simulink model "SingleTrack5states"  (R2018a)
settings: Solver=ode4  StartTime=0.0  StopTime=200  FixedStep=.001  MaxStep=0.001  MinStep=0.0001  RelTol=1e-1
values from neighbouring files (symbols this model uses):
  df_max = 0.35    [init_model.m]
  dr_max = 0    [init_model.m]
  initBeta = 0    [init_model.m]
  initR = 0    [init_model.m]
  initV = 10    [init_model.m]
  omegaR_max = 200    [init_model.m]
undefined symbols (not defined in the file or in its folder): car
settings Model: Creator=efrem  LastModifiedBy=efrem
settings SolverCC: ZeroCrossAlgorithm=Adaptive  AlgebraicLoopSolver=LineSearch
settings DebuggingCC: MaxConsecutiveZCsMsg=none
settings CodeAppCC: StateflowObjectComments=on

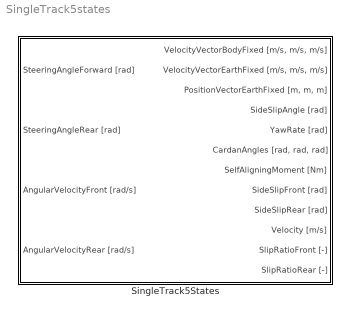
== system SingleTrack5states ==
  SingleTrack5States : Subsystem

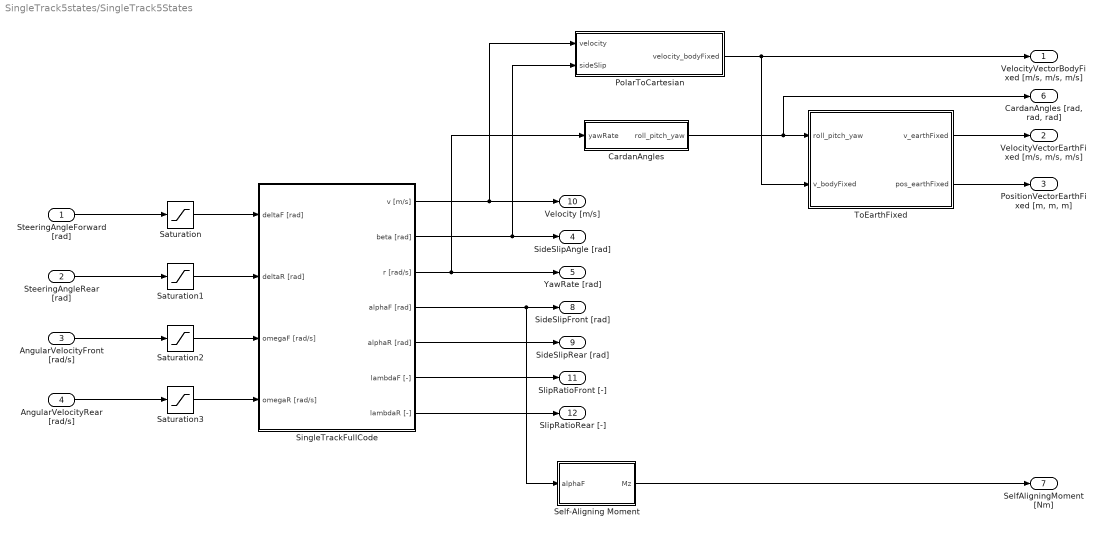
== system SingleTrack5states/SingleTrack5States ==
  SteeringAngleForward [rad] : Inport
  SteeringAngleRear [rad] : Inport  Port=2
  AngularVelocityFront [rad/s] : Inport  Port=3
  AngularVelocityRear [rad/s] : Inport  Port=4
  CardanAngles : Subsystem
  PolarToCartesian : Subsystem
  Saturation : Saturate  UpperLimit=df_max  LowerLimit=-df_max  ZeroCross=off
  Saturation1 : Saturate  UpperLimit=dr_max  LowerLimit=-dr_max  ZeroCross=off
  Saturation2 : Saturate  UpperLimit=omegaR_max  LowerLimit=0  ZeroCross=off
  Saturation3 : Saturate  UpperLimit=omegaR_max  LowerLimit=0  ZeroCross=off
  Self-Aligning Moment : Subsystem
  SingleTrackFullCode : Subsystem
  ToEarthFixed : Subsystem
  "VelocityVectorBodyFixed [m/s, m/s, m/s]" : Outport
  "VelocityVectorEarthFixed [m/s, m/s, m/s]" : Outport  Port=2
  "PositionVectorEarthFixed [m, m, m]" : Outport  Port=3
  SideSlipAngle [rad] : Outport  Port=4
  YawRate [rad] : Outport  Port=5
  "CardanAngles [rad, rad, rad]" : Outport  Port=6
  SelfAligningMoment [Nm] : Outport  Port=7
  SideSlipFront [rad] : Outport  Port=8
  SideSlipRear [rad] : Outport  Port=9
  Velocity [m/s] : Outport  Port=10
  SlipRatioFront [-] : Outport  Port=11
  SlipRatioRear [-] : Outport  Port=12
  wires:
  SingleTrackFullCode/3(r [rad/s]) -> CardanAngles/1(yawRate), YawRate [rad]/1
  ToEarthFixed/2(pos_earthFixed) -> "PositionVectorEarthFixed [m, m, m]"/1
  Self-Aligning Moment/1(Mz) -> SelfAligningMoment [Nm]/1
  PolarToCartesian/1(velocity_bodyFixed) -> ToEarthFixed/2(v_bodyFixed), "VelocityVectorBodyFixed [m/s, m/s, m/s]"/1
  SingleTrackFullCode/2(beta [rad]) -> PolarToCartesian/2(sideSlip), SideSlipAngle [rad]/1
  ToEarthFixed/1(v_earthFixed) -> "VelocityVectorEarthFixed [m/s, m/s, m/s]"/1
  CardanAngles/1(roll_pitch_yaw) -> ToEarthFixed/1(roll_pitch_yaw), "CardanAngles [rad, rad, rad]"/1
  SteeringAngleForward [rad]/1 -> Saturation/1
  AngularVelocityFront [rad/s]/1 -> Saturation2/1
  AngularVelocityRear [rad/s]/1 -> Saturation3/1
  Saturation1/1 -> SingleTrackFullCode/2(deltaR [rad])
  Saturation2/1 -> SingleTrackFullCode/3(omegaF [rad/s])
  Saturation3/1 -> SingleTrackFullCode/4(omegaR [rad/s])
  SteeringAngleRear [rad]/1 -> Saturation1/1
  SingleTrackFullCode/1(v [m/s]) -> PolarToCartesian/1(velocity), Velocity [m/s]/1
  Saturation/1 -> SingleTrackFullCode/1(deltaF [rad])
  SingleTrackFullCode/4(alphaF [rad]) -> Self-Aligning Moment/1(alphaF), SideSlipFront [rad]/1
  SingleTrackFullCode/5(alphaR [rad]) -> SideSlipRear [rad]/1
  SingleTrackFullCode/6(lambdaF [-]) -> SlipRatioFront [-]/1
  SingleTrackFullCode/7(lambdaR [-]) -> SlipRatioRear [-]/1

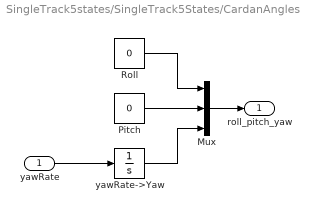
== system SingleTrack5states/SingleTrack5States/CardanAngles ==
  yawRate : Inport
  Mux : Mux  Inputs=3
  Pitch : Constant  Value=0
  Roll : Constant  Value=0
  yawRate->Yaw : Integrator
  roll_pitch_yaw : Outport
  wires:
  Pitch/1 -> Mux/2
  Roll/1 -> Mux/1
  Mux/1 -> roll_pitch_yaw/1
  yawRate->Yaw/1 -> Mux/3
  yawRate/1 -> yawRate->Yaw/1

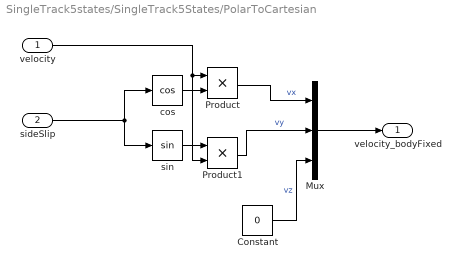
== system SingleTrack5states/SingleTrack5States/PolarToCartesian ==
  velocity : Inport
  sideSlip : Inport  Port=2
  Constant : Constant  Value=0
  Mux : Mux  Inputs=3
  Product : Product
  Product1 : Product
  cos : Trigonometry  Operator=cos
  sin : Trigonometry
  velocity_bodyFixed : Outport
  wires:
  Product/1 -> Mux/1  "vx"
  velocity/1 -> Product/1, Product1/2
  sin/1 -> Product1/1
  sideSlip/1 -> cos/1, sin/1
  Product1/1 -> Mux/2  "vy"
  cos/1 -> Product/2
  Constant/1 -> Mux/3  "vz"
  Mux/1 -> velocity_bodyFixed/1

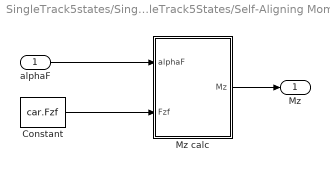
== system SingleTrack5states/SingleTrack5States/Self-Aligning Moment ==
  alphaF : Inport
  Constant : Constant  Value=car.Fzf
  Mz calc : MATLAB Function  TreatAsAtomicUnit=on
  Mz : Outport
  wires:
  Mz calc/1(Mz) -> Mz/1
  Constant/1 -> Mz calc/2(Fzf)
  alphaF/1 -> Mz calc/1(alphaF)

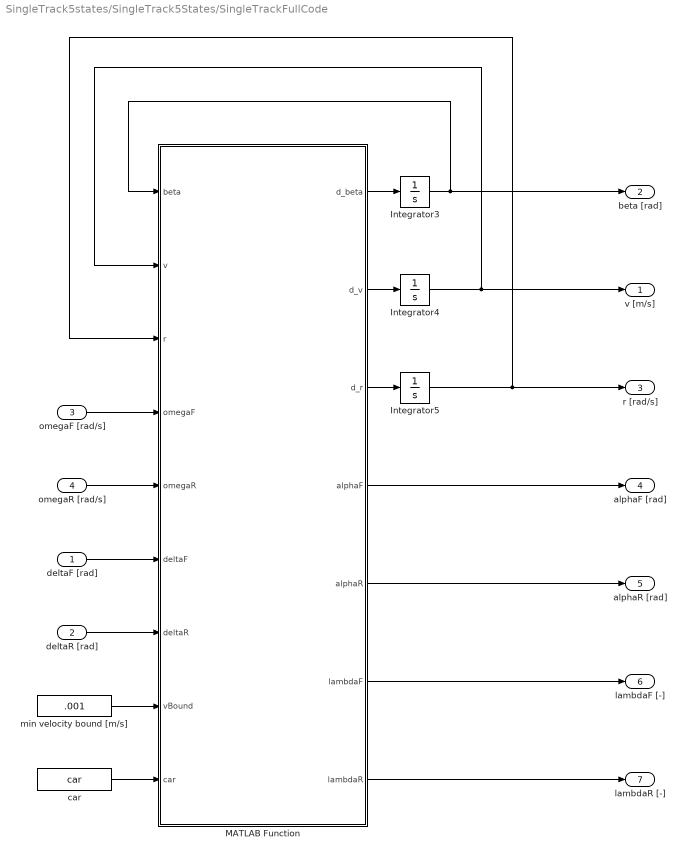
== system SingleTrack5states/SingleTrack5States/SingleTrackFullCode ==
  deltaF [rad] : Inport
  deltaR [rad] : Inport  Port=2
  omegaF [rad/s] : Inport  Port=3
  omegaR [rad/s] : Inport  Port=4
  Integrator3 : Integrator  InitialCondition=initBeta  UpperSaturationLimit=pi/2  LowerSaturationLimit=-pi/2  ZeroCross=off
  Integrator4 : Integrator  InitialCondition=initV  UpperSaturationLimit=pi/2  LowerSaturationLimit=-pi/2  ZeroCross=off
  Integrator5 : Integrator  InitialCondition=initR  UpperSaturationLimit=pi/2  LowerSaturationLimit=-pi/2  ZeroCross=off
  MATLAB Function : MATLAB Function  TreatAsAtomicUnit=on
  car : Constant  Value=car  OutDataTypeStr=Bus: car_bus
  min velocity bound [m/s] : Constant  Value=.001
  v [m/s] : Outport
  beta [rad] : Outport  Port=2
  r [rad/s] : Outport  Port=3
  alphaF [rad] : Outport  Port=4
  alphaR [rad] : Outport  Port=5
  lambdaF [-] : Outport  Port=6
  lambdaR [-] : Outport  Port=7
  wires:
  car/1 -> MATLAB Function/9(car)
  min velocity bound [m/s]/1 -> MATLAB Function/8(vBound)
  MATLAB Function/1(d_beta) -> Integrator3/1
  Integrator3/1 -> MATLAB Function/1(beta), beta [rad]/1
  MATLAB Function/2(d_v) -> Integrator4/1
  Integrator4/1 -> MATLAB Function/2(v), v [m/s]/1
  MATLAB Function/3(d_r) -> Integrator5/1
  Integrator5/1 -> MATLAB Function/3(r), r [rad/s]/1
  MATLAB Function/4(alphaF) -> alphaF [rad]/1
  MATLAB Function/5(alphaR) -> alphaR [rad]/1
  MATLAB Function/6(lambdaF) -> lambdaF [-]/1
  MATLAB Function/7(lambdaR) -> lambdaR [-]/1
  deltaF [rad]/1 -> MATLAB Function/6(deltaF)
  deltaR [rad]/1 -> MATLAB Function/7(deltaR)
  omegaF [rad/s]/1 -> MATLAB Function/4(omegaF)
  omegaR [rad/s]/1 -> MATLAB Function/5(omegaR)

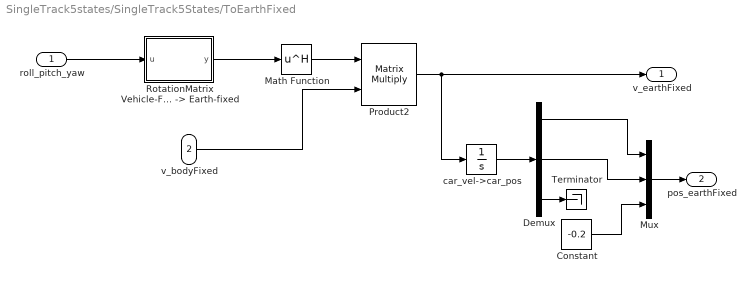
== system SingleTrack5states/SingleTrack5States/ToEarthFixed ==
  roll_pitch_yaw : Inport
  v_bodyFixed : Inport  Port=2
  Constant : Constant  Value=-0.2
  Demux : Demux  Outputs=3
  Math Function : Math  Operator=hermitian  SaturateOnIntegerOverflow=on
  Mux : Mux  Inputs=3
  Product2 : Product  Multiplication=Matrix(*)
  "RotationMatrix Vehicle-Fixed -> Earth-fixed" : MATLAB Function  TreatAsAtomicUnit=on
  Terminator : Terminator
  car_vel->car_pos : Integrator
  v_earthFixed : Outport
  pos_earthFixed : Outport  Port=2
  wires:
  v_bodyFixed/1 -> Product2/2
  Product2/1 -> v_earthFixed/1, car_vel->car_pos/1
  Constant/1 -> Mux/3
  Mux/1 -> pos_earthFixed/1
  car_vel->car_pos/1 -> Demux/1
  Demux/2 -> Mux/2
  Demux/1 -> Mux/1
  Math Function/1 -> Product2/1
  roll_pitch_yaw/1 -> "RotationMatrix Vehicle-Fixed -> Earth-fixed"/1(u)
  "RotationMatrix Vehicle-Fixed -> Earth-fixed"/1(y) -> Math Function/1
  Demux/3 -> Terminator/1

== matlab function SingleTrack5states/SingleTrack5States/ToEarthFixed/RotationMatrix Vehicle-Fixed -> Earth-fixed ==
  data: u input; y output
function y = fcn(u)

phi   = u(1); %roll
theta = u(2); %pitch
psi   = u(3); %yaw

% transformation matrix from the Earth-fixed to the vehicle-fixed
% coordinate frames
ETV = [cos(theta)*cos(psi),   sin(phi)*sin(theta)*cos(psi) - cos(phi)*sin(psi),   cos(phi)*sin(theta)*cos(psi) + sin(phi)*sin(psi);
       cos(theta)*sin(psi),   sin(phi)*sin(theta)*sin(psi) + cos(phi)*cos(psi),   cos(phi)*sin(theta)*sin(psi) - sin(phi)*cos(psi);
               -sin(theta),                                sin(phi)*cos(theta),                                cos(phi)*cos(theta)];
         
y = ETV';

== matlab function SingleTrack5states/SingleTrack5States/Self-Aligning Moment/Mz calc ==
  data: alphaF input; Mz output; Fzf input
function Mz = fcn(alphaF, Fzf)
    alphaF = rad2deg(alphaF);
    
    Bz = .15;
    Cz = 2.3;
    Dz = -.05 * Fzf;
    Ez = -10;
    
    Mz = Dz*sin((Cz*atan(Bz*alphaF - Ez*(Bz*alphaF - atan(Bz*alphaF)))));
end

== matlab function SingleTrack5states/SingleTrack5States/SingleTrackFullCode/MATLAB Function ==
  data: beta input; v input; r input; d_beta output; d_v output; d_r output; omegaF input; omegaR input; deltaF input; deltaR input; vBound input; car input; alphaF output; alphaR output; lambdaF output; lambdaR output
function [d_beta, d_v, d_r, alphaF, alphaR, lambdaF, lambdaR]= SingleTrackModel(beta, v, r, omegaF, omegaR, deltaF, deltaR, vBound, car)

    %% Parse Parameters 
    lf  = car.lf;
    lr  = car.lr;
    m   = car.m;
    Fzf = car.Fzf;
    Fzr = car.Fzr;
    p   = car.p;
    I   = car.I;
    
    Cdy = car.Tire.Cdy;
    Cby = car.Tire.Cby;
    Ccy = car.Tire.Ccy;
    Cey = car.Tire.Cey;
    Cdx = car.Tire.Cdx;
    Cbx = car.Tire.Cbx;
    Ccx = car.Tire.Ccx;
    Cex = car.Tire.Cex;
    
    %% Apply Deadzone for the Velocity (due to division by zero)
    if(v < vBound && v >= 0) 
		v = v+vBound;
	elseif (v > -vBound && v <0)
        v = v-vBound;
    end
    
    %% Wheel Kinematics
    vf = [cos(deltaF) sin(deltaF); -sin(deltaF) cos(deltaF)]*...
         [v*cos(beta); v*sin(beta) + lf*r];
    vr = [cos(deltaR) sin(deltaR); -sin(deltaR) cos(deltaR)]*...
         [v*cos(beta); v*sin(beta) - lr*r];
    vxf = vf(1);
    vyf = vf(2);
    vxr = vr(1);
    vyr = vr(2); 
    
    % slip angles of tires
    alphaF = -atan2(vyf, abs(vxf));
    alphaR = -atan2(vyr, abs(vxr));
     
    %% Slip Ratios
    lambdaF = (omegaF*p - vxf)/max(abs(omegaF*p), abs(vxf));
    lambdaR = (omegaR*p - vxr)/max(abs(omegaR*p), abs(vxr));
    
    lambdaF(lambdaF > 1)  = 1;
    lambdaF(lambdaF < -1) = -1;
    lambdaR(lambdaR > 1)  = 1;
    lambdaR(lambdaR < -1) = -1;
    
    %% Tire Models
    Fyf0 = Cdy * Fzf * sin(Ccy * atan(Cby*alphaF - Cey*(Cby*alphaF - atan(Cby*alphaF))));
    Fyr0 = Cdy * Fzr * sin(Ccy * atan(Cby*alphaR - Cey*(Cby*alphaR - atan(Cby*alphaR))));

    Fxf0 = Cdx * Fzf * sin(Ccx * atan(Cbx*lambdaF - Cex*(Cbx*lambdaF - atan(Cbx*lambdaF))));
    Fxr0 = Cdx * Fzr * sin(Ccx * atan(Cbx*lambdaR - Cex*(Cbx*lambdaR - atan(Cbx*lambdaR))));
    
    %% Traction Ellipse Front
    betaStar = acos(abs(lambdaF)/sqrt(lambdaF^2 + sin(alphaF)^2));

    mu_x_act = Fxf0/Fzf;
    mu_y_act = Fyf0/Fzf;

    mu_x_max = Cdx;
    mu_y_max = Cdy;

    mu_x = 1/sqrt((1/mu_x_act)^2 + (tan(betaStar)/mu_y_max)^2);
    mu_y = tan(betaStar)/sqrt((1/mu_x_max)^2 + (tan(betaStar)/mu_y_act)^2);

    Fxf = abs(mu_x/mu_x_act)*Fxf0;
    Fyf = abs(mu_y/mu_y_act)*Fyf0;

    if isnan(Fxf)
        Fxf = 0;
    end

    if isnan(Fyf)
        Fyf = 0;
    end

    if Fzf == 0
        Fxf = Fxf0;
        Fyf = Fyf0;
    end
    
    %% Traction Ellipse Rear
    betaStar = acos(abs(lambdaR)/sqrt(lambdaR^2 + sin(alphaR)^2));

    mu_x_act = Fxr0/Fzr;
    mu_y_act = Fyr0/Fzr;

    mu_x_max = Cdx;
    mu_y_max = Cdy;

    mu_x = 1/sqrt((1/mu_x_act)^2 + (tan(betaStar)/mu_y_max)^2);
    mu_y = tan(betaStar)/sqrt((1/mu_x_max)^2 + (tan(betaStar)/mu_y_act)^2);

    Fxr = abs(mu_x/mu_x_act)*Fxr0;
    Fyr = abs(mu_y/mu_y_act)*Fyr0;

    if isnan(Fxr)
        Fxr = 0;
    end

    if isnan(Fyr)
        Fyr = 0;
    end

    if Fzr == 0
        Fxr = Fxr0;
        Fyr = Fyr0;
    end
    
    %% Steering Angles Projection and Rigid Body Dynamics
    SAP = [cos(deltaF), -sin(deltaF), cos(deltaR), -sin(deltaR);...
        sin(deltaF), cos(deltaF), sin(deltaR), cos(deltaR);...
        lf*sin(deltaF), lf*cos(deltaF), -lr*sin(deltaR), -lr*cos(deltaR)];

    F = [Fxf; Fyf; Fxr; Fyr];

    RotDyn = [-sin(beta), cos(beta), 0;...
        cos(beta), sin(beta), 0;...
        0, 0, 1];
    
    C = diag([1/m/v, 1/m, 1/I]);
    
    Dyn = C * RotDyn * SAP * F - [r;0;0];
    
	%% Body states
    d_beta = Dyn(1);
    d_v    = Dyn(2);
    d_r    = Dyn(3); 

end
